simulink subsystem "Filtered_Derivative"  (R2019b)
settings: Solver=VariableStepAuto  StartTime=0.0  StopTime=10.0  RelTol=1e-3
model mask{num=[1 0], den=[1 0]}
  mask prompts: num "Numerator"; den "Denominator"
undefined symbols (not defined in the file): Anum, Bden, dt_control
settings Model: Creator=giaco  LastModifiedBy=alessandro

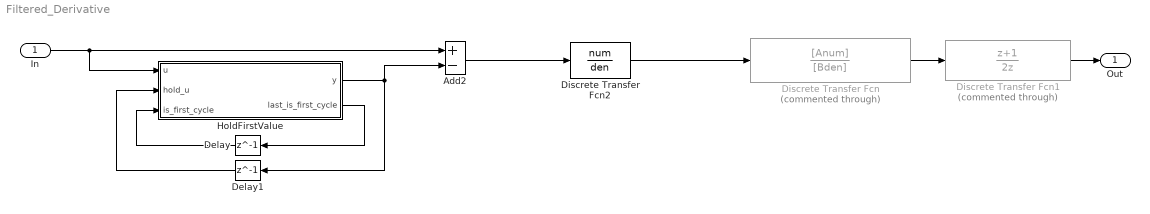
== system Filtered_Derivative ==
  In : Inport
  Add2 : Sum  Inputs=+-
  Delay : Delay  DelayLength=1  InitialCondition=1
  Delay1 : Delay  DelayLength=1  InitialCondition=1
  Discrete Transfer Fcn : DiscreteTransferFcn  Commented=through  Numerator=[Anum]  Denominator=[Bden]
  Discrete Transfer Fcn1 : DiscreteTransferFcn  Commented=through  Numerator=[1 1]  Denominator=[2 0]
  Discrete Transfer Fcn2 : DiscreteTransferFcn  Numerator=num  Denominator=den  SampleTime=dt_control
  HoldFirstValue : MATLAB Function  TreatAsAtomicUnit=on
  Out : Outport
  wires:
  Delay1/1 -> HoldFirstValue/2(hold_u)
  HoldFirstValue/2(last_is_first_cycle) -> Delay/1
  Delay/1 -> HoldFirstValue/3(is_first_cycle)
  Add2/1 -> Discrete Transfer Fcn2/1
  HoldFirstValue/1(y) -> Delay1/1, Add2/2
  Discrete Transfer Fcn2/1 -> Discrete Transfer Fcn/1
  In/1 -> Add2/1, HoldFirstValue/1(u)
  Discrete Transfer Fcn/1 -> Discrete Transfer Fcn1/1
  Discrete Transfer Fcn1/1 -> Out/1

== matlab function Filtered_Derivative/HoldFirstValue ==
  data: u input; y output; hold_u input; is_first_cycle input; last_is_first_cycle output
function [y,last_is_first_cycle]  = holdFirstValue(u, hold_u, is_first_cycle)

if is_first_cycle
    y = u;
else
    y = hold_u;
end
last_is_first_cycle = 0;

end
